simulink model "MdXX_IsStBsy"  (R2018b)
settings: Solver=FixedStepDiscrete  StartTime=0.0  StopTime=10.0  FixedStep=0.01  RelTol=1e-3
settings Model: Creator=sn2xws  LastModifiedBy=sn2xws
settings DataIOCC: SaveFormat=StructureWithTime
settings OptimizationCC: DefaultParameterBehavior=Inlined  EnhancedBackFolding=on  PassReuseOutputArgsAs=Individual arguments  ZeroExternalMemoryAtStartup=off  ZeroInternalMemoryAtStartup=off  OptimizeBlockOrder=speed  DifferentSizesBufferReuse=on  OptimizationCustomize=off
settings DebuggingCC: ParameterTunabilityLossMsg=error
settings ModelReferenceCC: ModelReferenceNumInstancesAllowed=Single
settings SFSimCC: MATLABDynamicMemAlloc=off
settings RTWCC: SystemTargetFile=autosar.tlc  GenCodeOnly=on  TemplateMakefile=ert_default_tmf  Description=AUTOSAR  GenerateReport=on  IncludeHyperlinkInReport=on  LaunchReport=on  GenerateTraceInfo=on  GenerateTraceReport=on  GenerateTraceReportSl=on  GenerateTraceReportSf=on  GenerateTraceReportEml=on
settings CodeAppCC: ForceParamTrailComments=on  IgnoreCustomStorageClasses=off  OperatorAnnotations=on  SimulinkDataObjDesc=on  SFDataObjDesc=on  InsertBlockDesc=on
settings STFCustomTargetCC: TargetLangStandard=C99 (ISO)  MultiwordLength=256  ParMdlRefBuildCompliant=on  CompOptLevelCompliant=on  IncludeMdlTerminateFcn=off  CombineOutputUpdateFcns=on  SuppressErrorStatus=on  ERTCustomFileBanners=on  SupportNonFinite=off  SupportComplex=off  SupportContinuousTime=off  SupportNonInlinedSFcns=off  RemoveResetFunc=on  MATLABClassNameForMDSCustomization=Simulink.SoftwareTarget.ERTCustomization  AutosarCompliant=on  UseToolchainInfoCompliant=on  LookupTableObjectStructAxisOrder=2,1,3,4,...  LUTObjectStructOrderEvenSpacing=Size,Table,Breakpoints  SystemTargetFile=autosar.tlc
settings ERTTargetCC: TargetLangStandard=C99 (ISO)  ConcurrentExecutionCompliant=off  IncludeMdlTerminateFcn=off  SuppressErrorStatus=on  SupportNonFinite=off  SupportComplex=off  ModelStepFunctionPrototypeControlCompliant=off  CPPClassGenCompliant=off  AutosarCompliant=on  LookupTableObjectStructAxisOrder=2,1,3,4,...  LUTObjectStructOrderEvenSpacing=Size,Table,Breakpoints  InlinedParameterPlacement=NonHierarchical  ERTCustomFileTemplate=example_file_process.tlc

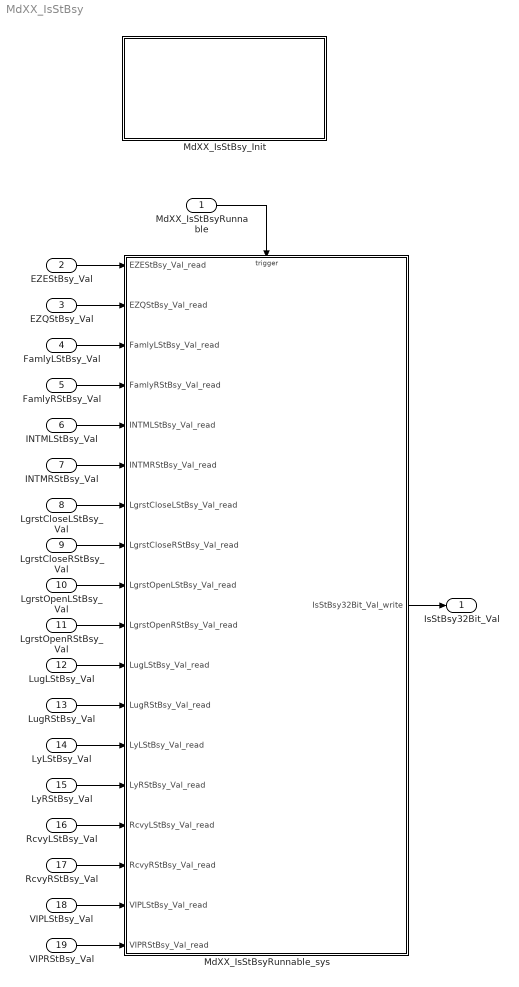
== system MdXX_IsStBsy ==
  MdXX_IsStBsyRunnable : Inport  SampleTime=0.01  OutputFunctionCall=on
  EZEStBsy_Val : Inport  Port=2  OutDataTypeStr=boolean  PortDimensions=1
  EZQStBsy_Val : Inport  Port=3  OutDataTypeStr=boolean  PortDimensions=1
  FamlyLStBsy_Val : Inport  Port=4  OutDataTypeStr=boolean  PortDimensions=1
  FamlyRStBsy_Val : Inport  Port=5  OutDataTypeStr=boolean  PortDimensions=1
  INTMLStBsy_Val : Inport  Port=6  OutDataTypeStr=boolean  PortDimensions=1
  INTMRStBsy_Val : Inport  Port=7  OutDataTypeStr=boolean  PortDimensions=1
  LgrstCloseLStBsy_Val : Inport  Port=8  OutDataTypeStr=boolean  PortDimensions=1
  LgrstCloseRStBsy_Val : Inport  Port=9  OutDataTypeStr=boolean  PortDimensions=1
  LgrstOpenLStBsy_Val : Inport  Port=10  OutDataTypeStr=boolean  PortDimensions=1
  LgrstOpenRStBsy_Val : Inport  Port=11  OutDataTypeStr=boolean  PortDimensions=1
  LugLStBsy_Val : Inport  Port=12  OutDataTypeStr=boolean  PortDimensions=1
  LugRStBsy_Val : Inport  Port=13  OutDataTypeStr=boolean  PortDimensions=1
  LyLStBsy_Val : Inport  Port=14  OutDataTypeStr=boolean  PortDimensions=1
  LyRStBsy_Val : Inport  Port=15  OutDataTypeStr=boolean  PortDimensions=1
  RcvyLStBsy_Val : Inport  Port=16  OutDataTypeStr=boolean  PortDimensions=1
  RcvyRStBsy_Val : Inport  Port=17  OutDataTypeStr=boolean  PortDimensions=1
  VIPLStBsy_Val : Inport  Port=18  OutDataTypeStr=boolean  PortDimensions=1
  VIPRStBsy_Val : Inport  Port=19  OutDataTypeStr=boolean  PortDimensions=1
  MdXX_IsStBsyRunnable_sys : Subsystem
  MdXX_IsStBsy_Init : Subsystem
  IsStBsy32Bit_Val : Outport  OutDataTypeStr=uint32  PortDimensions=1
  wires:
  EZEStBsy_Val/1 -> MdXX_IsStBsyRunnable_sys/1(EZEStBsy_Val_read)
  EZQStBsy_Val/1 -> MdXX_IsStBsyRunnable_sys/2(EZQStBsy_Val_read)
  FamlyLStBsy_Val/1 -> MdXX_IsStBsyRunnable_sys/3(FamlyLStBsy_Val_read)
  FamlyRStBsy_Val/1 -> MdXX_IsStBsyRunnable_sys/4(FamlyRStBsy_Val_read)
  INTMLStBsy_Val/1 -> MdXX_IsStBsyRunnable_sys/5(INTMLStBsy_Val_read)
  INTMRStBsy_Val/1 -> MdXX_IsStBsyRunnable_sys/6(INTMRStBsy_Val_read)
  LgrstCloseLStBsy_Val/1 -> MdXX_IsStBsyRunnable_sys/7(LgrstCloseLStBsy_Val_read)
  LgrstCloseRStBsy_Val/1 -> MdXX_IsStBsyRunnable_sys/8(LgrstCloseRStBsy_Val_read)
  LgrstOpenLStBsy_Val/1 -> MdXX_IsStBsyRunnable_sys/9(LgrstOpenLStBsy_Val_read)
  LgrstOpenRStBsy_Val/1 -> MdXX_IsStBsyRunnable_sys/10(LgrstOpenRStBsy_Val_read)
  LugLStBsy_Val/1 -> MdXX_IsStBsyRunnable_sys/11(LugLStBsy_Val_read)
  LugRStBsy_Val/1 -> MdXX_IsStBsyRunnable_sys/12(LugRStBsy_Val_read)
  LyLStBsy_Val/1 -> MdXX_IsStBsyRunnable_sys/13(LyLStBsy_Val_read)
  LyRStBsy_Val/1 -> MdXX_IsStBsyRunnable_sys/14(LyRStBsy_Val_read)
  RcvyLStBsy_Val/1 -> MdXX_IsStBsyRunnable_sys/15(RcvyLStBsy_Val_read)
  RcvyRStBsy_Val/1 -> MdXX_IsStBsyRunnable_sys/16(RcvyRStBsy_Val_read)
  VIPLStBsy_Val/1 -> MdXX_IsStBsyRunnable_sys/17(VIPLStBsy_Val_read)
  VIPRStBsy_Val/1 -> MdXX_IsStBsyRunnable_sys/18(VIPRStBsy_Val_read)
  MdXX_IsStBsyRunnable_sys/1(IsStBsy32Bit_Val_write) -> IsStBsy32Bit_Val/1
  MdXX_IsStBsyRunnable/1 -> MdXX_IsStBsyRunnable_sys/Trigger

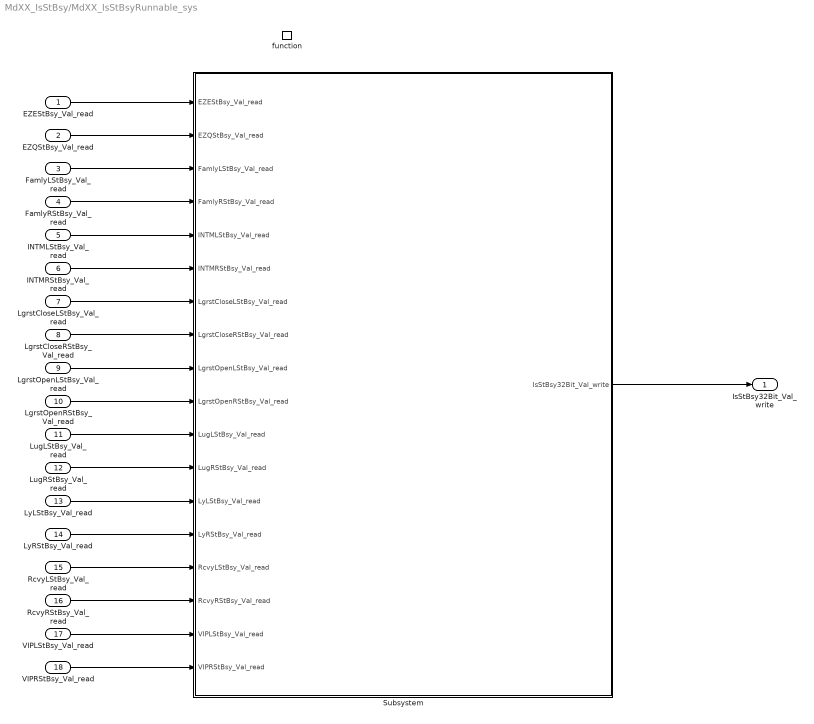
== system MdXX_IsStBsy/MdXX_IsStBsyRunnable_sys ==
  EZEStBsy_Val_read : Inport
  EZQStBsy_Val_read : Inport  Port=2
  FamlyLStBsy_Val_read : Inport  Port=3
  FamlyRStBsy_Val_read : Inport  Port=4
  INTMLStBsy_Val_read : Inport  Port=5
  INTMRStBsy_Val_read : Inport  Port=6
  LgrstCloseLStBsy_Val_read : Inport  Port=7
  LgrstCloseRStBsy_Val_read : Inport  Port=8
  LgrstOpenLStBsy_Val_read : Inport  Port=9
  LgrstOpenRStBsy_Val_read : Inport  Port=10
  LugLStBsy_Val_read : Inport  Port=11
  LugRStBsy_Val_read : Inport  Port=12
  LyLStBsy_Val_read : Inport  Port=13
  LyRStBsy_Val_read : Inport  Port=14
  RcvyLStBsy_Val_read : Inport  Port=15
  RcvyRStBsy_Val_read : Inport  Port=16
  VIPLStBsy_Val_read : Inport  Port=17
  VIPRStBsy_Val_read : Inport  Port=18
  function : TriggerPort  TriggerType=function-call  VariantControl=(inherit)  SampleTimeType=periodic  SampleTime=-1
  Subsystem : Subsystem
  IsStBsy32Bit_Val_write : Outport
      settings: EnsureOutportIsVirtual=on
  wires:
  EZEStBsy_Val_read/1 -> Subsystem/1(EZEStBsy_Val_read)
  EZQStBsy_Val_read/1 -> Subsystem/2(EZQStBsy_Val_read)
  FamlyLStBsy_Val_read/1 -> Subsystem/3(FamlyLStBsy_Val_read)
  FamlyRStBsy_Val_read/1 -> Subsystem/4(FamlyRStBsy_Val_read)
  INTMLStBsy_Val_read/1 -> Subsystem/5(INTMLStBsy_Val_read)
  INTMRStBsy_Val_read/1 -> Subsystem/6(INTMRStBsy_Val_read)
  LgrstCloseLStBsy_Val_read/1 -> Subsystem/7(LgrstCloseLStBsy_Val_read)
  LgrstCloseRStBsy_Val_read/1 -> Subsystem/8(LgrstCloseRStBsy_Val_read)
  LgrstOpenLStBsy_Val_read/1 -> Subsystem/9(LgrstOpenLStBsy_Val_read)
  LgrstOpenRStBsy_Val_read/1 -> Subsystem/10(LgrstOpenRStBsy_Val_read)
  LugLStBsy_Val_read/1 -> Subsystem/11(LugLStBsy_Val_read)
  LugRStBsy_Val_read/1 -> Subsystem/12(LugRStBsy_Val_read)
  LyLStBsy_Val_read/1 -> Subsystem/13(LyLStBsy_Val_read)
  LyRStBsy_Val_read/1 -> Subsystem/14(LyRStBsy_Val_read)
  RcvyLStBsy_Val_read/1 -> Subsystem/15(RcvyLStBsy_Val_read)
  RcvyRStBsy_Val_read/1 -> Subsystem/16(RcvyRStBsy_Val_read)
  VIPLStBsy_Val_read/1 -> Subsystem/17(VIPLStBsy_Val_read)
  VIPRStBsy_Val_read/1 -> Subsystem/18(VIPRStBsy_Val_read)
  Subsystem/1(IsStBsy32Bit_Val_write) -> IsStBsy32Bit_Val_write/1

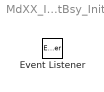
== system MdXX_IsStBsy/MdXX_IsStBsy_Init ==
  Event Listener : EventListener  EventName=reset

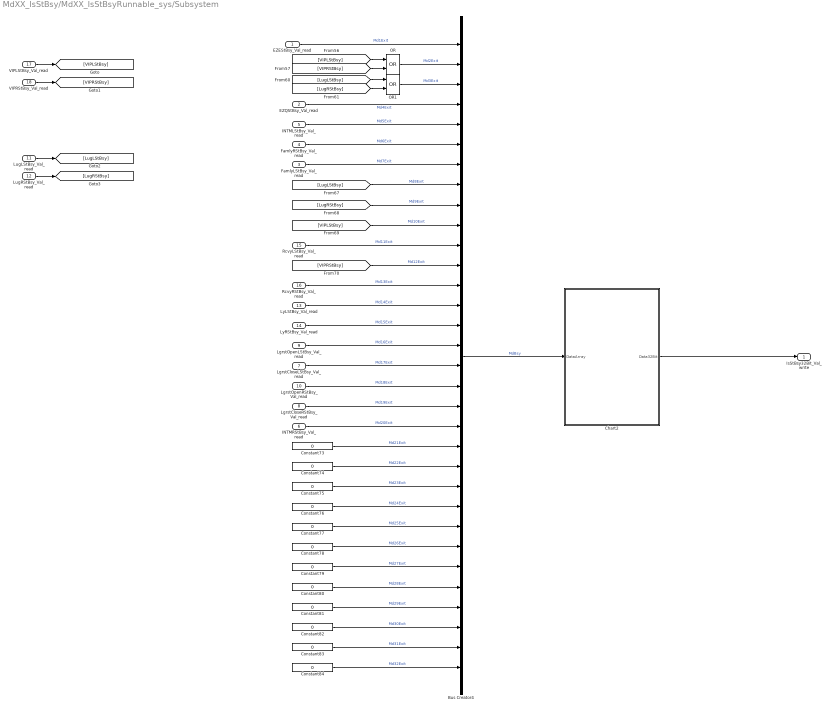
== system MdXX_IsStBsy/MdXX_IsStBsyRunnable_sys/Subsystem ==
  EZEStBsy_Val_read : Inport
  EZQStBsy_Val_read : Inport  Port=2
  FamlyLStBsy_Val_read : Inport  Port=3
  FamlyRStBsy_Val_read : Inport  Port=4
  INTMLStBsy_Val_read : Inport  Port=5
  INTMRStBsy_Val_read : Inport  Port=6
  LgrstCloseLStBsy_Val_read : Inport  Port=7
  LgrstCloseRStBsy_Val_read : Inport  Port=8
  LgrstOpenLStBsy_Val_read : Inport  Port=9
  LgrstOpenRStBsy_Val_read : Inport  Port=10
  LugLStBsy_Val_read : Inport  Port=11
  LugRStBsy_Val_read : Inport  Port=12
  LyLStBsy_Val_read : Inport  Port=13
  LyRStBsy_Val_read : Inport  Port=14
  RcvyLStBsy_Val_read : Inport  Port=15
  RcvyRStBsy_Val_read : Inport  Port=16
  VIPLStBsy_Val_read : Inport  Port=17
  VIPRStBsy_Val_read : Inport  Port=18
  Bus Creator4 : BusCreator  Inputs=32
  Chart2 : Stateflow chart  TreatAsAtomicUnit=on
  Constant{73..84} (12 alike) : Constant  Value=0  OutDataTypeStr=boolean
  OR : Logic  Operator=OR  AllPortsSameDT=off  OutDataTypeStr=boolean
  OR1 : Logic  Operator=OR  AllPortsSameDT=off  OutDataTypeStr=boolean
  IsStBsy32Bit_Val_write : Outport
      settings: EnsureOutportIsVirtual=on
  wires:
  [VIPLStBsy] -> OR/1
  RcvyLStBsy_Val_read/1 -> Bus Creator4/11  "Md11Exit"
  [LugLStBsy] -> OR1/1
  LgrstOpenLStBsy_Val_read/1 -> Bus Creator4/16  "Md16Exit"
  Constant78/1 -> Bus Creator4/26  "Md26Exit"
  [VIPRStBsy] -> OR/2
  Constant74/1 -> Bus Creator4/22  "Md22Exit"
  RcvyRStBsy_Val_read/1 -> Bus Creator4/13  "Md13Exit"
  EZQStBsy_Val_read/1 -> Bus Creator4/4  "Md4Exit"
  Constant73/1 -> Bus Creator4/21  "Md21Exit"
  [LugRStBsy] -> OR1/2
  [LugRStBsy] -> Bus Creator4/9  "Md9Exit"
  INTMLStBsy_Val_read/1 -> Bus Creator4/5  "Md5Exit"
  OR/1 -> Bus Creator4/2  "Md2Exit"
  Constant84/1 -> Bus Creator4/32  "Md32Exit"
  FamlyLStBsy_Val_read/1 -> Bus Creator4/7  "Md7Exit"
  OR1/1 -> Bus Creator4/3  "Md3Exit"
  Constant77/1 -> Bus Creator4/25  "Md25Exit"
  LgrstCloseLStBsy_Val_read/1 -> Bus Creator4/17  "Md17Exit"
  [VIPRStBsy] -> Bus Creator4/12  "Md12Exit"
  LgrstOpenRStBsy_Val_read/1 -> Bus Creator4/18  "Md18Exit"
  Bus Creator4/1 -> Chart2/1(DataArray)  "MdBsy"
  INTMRStBsy_Val_read/1 -> Bus Creator4/20  "Md20Exit"
  LgrstCloseRStBsy_Val_read/1 -> Bus Creator4/19  "Md19Exit"
  LyLStBsy_Val_read/1 -> Bus Creator4/14  "Md14Exit"
  Constant82/1 -> Bus Creator4/30  "Md30Exit"
  Constant83/1 -> Bus Creator4/31  "Md31Exit"
  EZEStBsy_Val_read/1 -> Bus Creator4/1  "Md1Exit"
  [LugLStBsy] -> Bus Creator4/8  "Md8Exit"
  FamlyRStBsy_Val_read/1 -> Bus Creator4/6  "Md6Exit"
  Constant75/1 -> Bus Creator4/23  "Md23Exit"
  Constant79/1 -> Bus Creator4/27  "Md27Exit"
  [VIPLStBsy] -> Bus Creator4/10  "Md10Exit"
  Constant80/1 -> Bus Creator4/28  "Md28Exit"
  Constant76/1 -> Bus Creator4/24  "Md24Exit"
  Constant81/1 -> Bus Creator4/29  "Md29Exit"
  LyRStBsy_Val_read/1 -> Bus Creator4/15  "Md15Exit"
  Chart2/1(Data32Bit) -> IsStBsy32Bit_Val_write/1
  VIPLStBsy_Val_read/1 -> [VIPLStBsy]
  VIPRStBsy_Val_read/1 -> [VIPRStBsy]
  LugLStBsy_Val_read/1 -> [LugLStBsy]
  LugRStBsy_Val_read/1 -> [LugRStBsy]

== stateflow chart MdXX_IsStBsy/MdXX_IsStBsyRunnable_sys/Subsystem/Chart2 ==
  (default) -> (junction 3) : {Data32Bit = 0x00000000;}
  (junction 3) -> (junction 9) : {i = 0;}
  (junction 9) -> (junction 4) [order 1] : [i < 32]
  (junction 4) -> (junction 1) : {
      | temp_var = uint32(DataArray[i]);
      | temp_var= temp_var << i;
      | Data32Bit = Data32Bit |  temp_var;
      | }
  (junction 1) -> (junction 9) : {i++;}
  (junction 9) -> (junction 5) [order 2]
  data: Data32Bit output uint32; DataArray input boolean size=32; temp_var local uint32; i local uint8
